simulink model "A1_Servoventil_Test"  (Simulink 8.7)
settings: Solver=ode4  StartTime=0.0  StopTime=10.0  FixedStep=1e-3  RelTol=1e-3
libraries: simulink x1
settings Model: Creator=jinyao  LastModifiedBy=jinyao
settings DataIOCC: LimitDataPoints=off  SaveFormat=Dataset
settings DebuggingCC: UnderspecifiedInitializationDetection=Simplified  MergeDetectMultiDrivingBlocksExec=error
settings HardwareCC: ProdBitPerPointer=64  ProdLargestAtomicFloat=Float  ProdIntDivRoundTo=Zero  ProdEndianess=LittleEndian  ProdWordSize=64  ProdHWDeviceType=Intel->x86-64 (Windows64)
settings ModelReferenceCC: PropagateSignalLabelsOutOfModel=on
settings ConfigComp: CovModelRefEnable=off

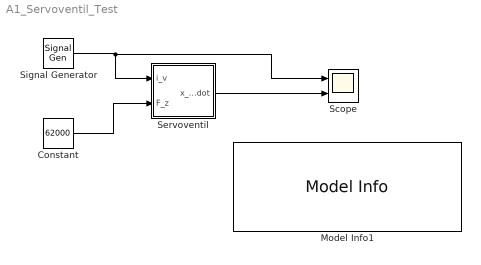
== system A1_Servoventil_Test ==
  Constant : Constant  Value=62000
  Model Info1 : simulink/Model-Wide Utilities/Model Info  Frame=on  DisplayStringWithTags=|  HorizontalTextAlignment=Center  LeftAlignmentValue=0.5  SourceBlockDiagram=A1_Servoventil_Test  TagMaxNumber=20
      | %<ModelName>
      | 
      | MODSIM GRUPPE 11
      | 
      | Cao,Bozhi  Gao,Yue  Jia,Xuehua  Zhu,Jinyao
      | 
      | 14.06.2018
  Scope : Scope  NumInputPorts=2
  Servoventil : Subsystem
  Signal Generator : SignalGenerator  Amplitude=2  Frequency=2  Units=rad/sec
  wires:
  Constant/1 -> Servoventil/2(F_z)
  Signal Generator/1 -> Scope/1, Servoventil/1(i_v)
  Servoventil/1(x_oil_dot) -> Scope/2

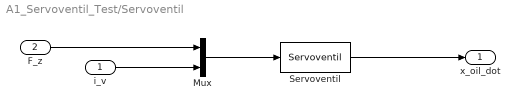
== system A1_Servoventil_Test/Servoventil ==
  i_v : Inport
  F_z : Inport  Port=2
  Mux : Mux  Inputs=2
  Servoventil : MATLABFcn  MATLABFcn=Servoventil  OutputDimensions=1  OutputSignalType=real
  x_oil_dot : Outport
  wires:
  Servoventil/1 -> x_oil_dot/1
  i_v/1 -> Mux/2
  Mux/1 -> Servoventil/1
  F_z/1 -> Mux/1
